simulink model "untitled"  (R2022a)
settings: Solver=FixedStepDiscrete  StartTime=0.0  StopTime=10.0  FixedStep=0.001  RelTol=1e-3
undefined symbols (not defined in the file): DiscIntNeverNeededParam
libraries: GPIO_Lib x8, TIMERS_Lib x8, CAN_Lib x7, USART_Lib x3, STM32_Config_Lib x1
settings Model: Creator=Administrator  LastModifiedBy=Administrator
settings SolverCC: AutoInsertRateTranBlk=on
settings OptimizationCC: DefaultParameterBehavior=Inlined  EnhancedBackFolding=on  PassReuseOutputArgsAs=Individual arguments  ZeroExternalMemoryAtStartup=off  ZeroInternalMemoryAtStartup=off  OptimizeBlockOrder=speed  DifferentSizesBufferReuse=on  OptimizationCustomize=off  EfficientTunableParamExpr=on
settings DebuggingCC: MultiTaskDSMMsg=none  ParameterTunabilityLossMsg=error
settings HardwareCC: ProdBitPerPointer=32  ProdBitPerSizeT=32  ProdBitPerPtrDiffT=32  ProdLargestAtomicInteger=Long  ProdLargestAtomicFloat=Double  ProdWordSize=32  ProdHWDeviceType=ARM Compatible->ARM Cortex-M
settings SFSimCC: MATLABDynamicMemAlloc=off
settings RTWCC: Description=stm32 (Embedded Target)  SystemTargetFile=stm32.tlc  TemplateMakefile=stm32.tmf  GenerateReport=on
settings RTWCC: CustomHeaderCode=|
  | #include "untitled_private.h"
  | #include "string.h"
  | #include "math.h"
settings CodeAppCC: ForceParamTrailComments=on  IgnoreCustomStorageClasses=off  MaxIdLength=64  OperatorAnnotations=on  SimulinkDataObjDesc=on  SFDataObjDesc=on  CustomSymbolStrType=$N$R$M  SimulinkBlockComments=off
settings STFCustomTargetCC: TargetLangStandard=C99 (ISO)  CodeReplacementLibrary=ARM CMSIS SIN COS  MultiwordLength=256  ParMdlRefBuildCompliant=on  IncludeMdlTerminateFcn=off  CombineOutputUpdateFcns=on  ERTCustomFileBanners=on  SupportNonInlinedSFcns=off  RemoveResetFunc=on  MATLABClassNameForMDSCustomization=Simulink.SoftwareTarget.ERTCustomization  GRTInterface=off  SystemTargetFile=stm32.tlc
settings ERTTargetCC: TargetLangStandard=C99 (ISO)  CodeReplacementLibrary=ARM CMSIS SIN COS  CompOptLevelCompliant=off  ConcurrentExecutionCompliant=off  IncludeMdlTerminateFcn=off  SupportContinuousTime=on  ModelStepFunctionPrototypeControlCompliant=off  CPPClassGenCompliant=off  UseToolchainInfoCompliant=off  ExtModeStaticAllocSize=256  ExtModeMexFile=ext_serial_win32_comm  ExtModeMexArgs=0,1,115200,10  InlinedParameterPlacement=NonHierarchical  ERTSrcFileBannerTemplate=sourceFileTemplate.cgt  ERTHdrFileBannerTemplate=sourceFileTemplate.cgt  ERTDataSrcFileTemplate=sourceFileTemplate.cgt  ERTDataHdrFileTemplate=sourceFileTemplate.cgt  ERTCustomFileTemplate=customRoutineProcess.tlc

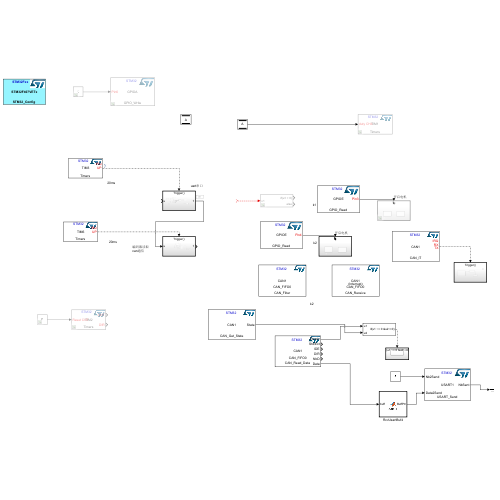
[thumbnail: Simulink's stored preview of the top-level diagram]
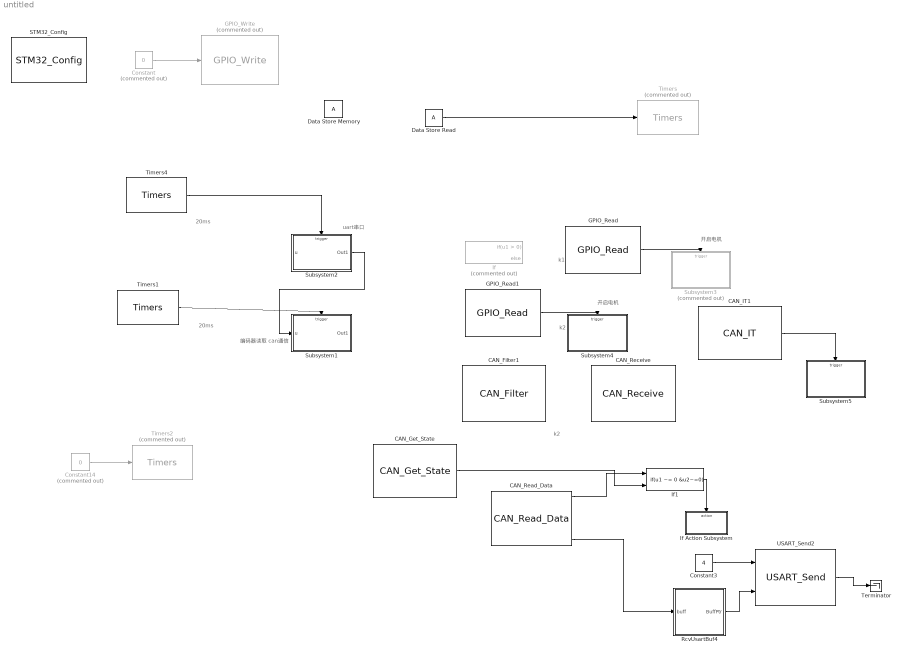
== system untitled ==
  note: 开启电机
  note: uart串口
  note: 编码器读取
      | can通信
  note: 20ms
  note: 20ms
  note: k2
  note: k1
  note: k2
  note: 开启电机
  CAN_Filter1 : CAN_Lib/CAN_Filter  CAN_name=CAN1  CAN_Filter_Activation=on  CAN_Filter_Scale=CAN_FILTERSCALE_16BIT  CAN_Filter_Mask_Id_High=0  CAN_Filter_Mask_Id_Low=0  CAN_Filter_Id_High=0  CAN_Filter_Id_Low=0  CAN_Filter_FIFO_Assignment=CAN_FIFO0  CAN_Filter_Bank=0  CAN_Filter_Mode=CAN_FILTERMODE_IDMASK  CAN_Filter_Slave_Start_Bank=14
      settings: SourceProductName=Target Support Package - STM32 Adapter
  CAN_Get_State : CAN_Lib/CAN_Get_State  CAN_name=CAN1
      settings: SourceProductName=Target Support Package - STM32 Adapter
  CAN_IT1 : CAN_Lib/CAN_IT  CAN_name=CAN1  CAN_Mode=Master  CAN_It=on  CAN_RX_It=on  CAN_TX_It=on  CAN_ERROR_It=off
      settings: SourceProductName=Target Support Package - STM32 Adapter
  CAN_Read_Data : CAN_Lib/CAN_Read_Data  CAN_name=CAN1  CAN_Fifo=CAN_FIFO0  CAN_MsgType=off
      settings: SourceProductName=Target Support Package - STM32 Adapter
  CAN_Receive : CAN_Lib/CAN_Receive  CAN_name=CAN1  CAN_Mode=Master  CAN_It=on  CAN_Fifo=CAN_FIFO0
      settings: SourceProductName=Target Support Package - STM32 Adapter
  Constant : Constant  Commented=on  Value=0
  Constant14 : Constant  Commented=on  Value=0  OutDataTypeStr=uint16
  Constant3 : Constant  Value=4  OutDataTypeStr=uint16
  Data Store Memory : DataStoreMemory  WriteAfterWriteMsg=warning  ShowAdditionalParam=off
  Data Store Read : DataStoreRead  IndexOptions=Index vector (dialog)  Indices=1  OutputSizes=1
  GPIO_Read : GPIO_Lib/GPIO_Read  Port_name=GPIOE  Pin_0=off  Pin_1=off  Pin_2=off  Pin_3=on  Pin_4=off  Pin_5=off  Pin_6=off  Pin_7=off  Pin_8=off  Pin_9=off  Pin_10=off  Pin_11=off  Pin_12=off  Pin_13=off  Pin_14=off  Pin_15=off  PinList="GPIOE3  4"
      settings: SourceProductName=Target Support Package - STM32 Adapter
  GPIO_Read1 : GPIO_Lib/GPIO_Read  Port_name=GPIOE  Pin_0=off  Pin_1=off  Pin_2=off  Pin_3=off  Pin_4=on  Pin_5=off  Pin_6=off  Pin_7=off  Pin_8=off  Pin_9=off  Pin_10=off  Pin_11=off  Pin_12=off  Pin_13=off  Pin_14=off  Pin_15=off  PinList="GPIOE3  4"
      settings: SourceProductName=Target Support Package - STM32 Adapter
  GPIO_Write : GPIO_Lib/GPIO_Write  Commented=on  Port_name=GPIOA  Pin0=off  Toggle_Pin0=off  Pin1=off  Toggle_Pin1=off  Pin2=off  Toggle_Pin2=off  Pin3=off  Toggle_Pin3=off  Pin4=off  Toggle_Pin4=off  Pin5=off  Toggle_Pin5=off  Pin6=on  Toggle_Pin6=off  Pin7=off  Toggle_Pin7=off  Pin8=off  Toggle_Pin8=off  Pin9=off  Toggle_Pin9=off  Pin10=off  Toggle_Pin10=off  Pin11=off  Toggle_Pin11=off  Pin12=off  Toggle_Pin12=off  Pin13=off  Toggle_Pin13=off  Pin14=off  Toggle_Pin14=off  Pin15=off  Toggle_Pin15=off  PinList="GPIOA6  7GPIOE13"
      settings: SourceProductName=Target Support Package - STM32 Adapter
  If : If  Commented=on
  If Action Subsystem : Subsystem  TreatAsAtomicUnit=on
  If1 : If  NumInputs=2  IfExpression=u1 ~= 0 &u2~=0  ShowElse=off
  RcvUsartBuf4 : MATLAB Function  TreatAsAtomicUnit=on
  STM32_Config : STM32_Config_Lib/STM32_Config  Priority=0  Project_Path=C:\Users\Administrator\Desktop\bishe\  Config_File=bishe.ioc  MCU_Name=STM32F407VETx
      settings: SourceProductName=Target Support Package - STM32 Adapter
  Subsystem1 : Subsystem
  Subsystem2 : Subsystem
  Subsystem3 : Subsystem  Commented=on
  Subsystem4 : Subsystem
  Subsystem5 : Subsystem
  Terminator : Terminator
  Timers : TIMERS_Lib/Timers  Commented=on  currentTIM=TIM1  TIM_Name=TIM1  sysUsingTimer=off  TIM_APBClock=168000000  TIM_Set_Clk=off  TIM_Prescaler=1000-1  TIM_Clock=168000.00  Variable_frequency=off  TIM_Set_OutFreq=off  TIM_ARR=1  Output_frequency=168000.00  Repetition_counter=0  TIM_Mode=Up  TIM_DMA=none  TIM_IRQ=on  TIM_IRQ_ONLY=off  TIM_UP=off  TIM_TRG=off  TIM_COM=off  TIM_BRK=off  NbTIM=5  CH1_enable=off  CH1N_enable=off  CH1_type=Unknown  CH1_DMA=off  CH1_int=off  CH1_edge=Rising  CH1_div=1  CH1_variable_duty=off  CH1_set_pulse=off  CH1_output_duty=0.00  CH1_pulse=0  CH2_enable=off  CH2N_enable=off  CH2_type=Unknown  CH2_DMA=off  CH2_int=off  CH2_edge=Rising  CH2_div=1  CH2_variable_duty=off  CH2_set_pulse=off  CH2_output_duty=0.00  CH2_pulse=0  CH3_enable=off  CH3N_enable=off  CH3_type=Unknown  CH3_DMA=off  CH3_int=off  CH3_edge=Rising  CH3_div=1  CH3_variable_duty=off  CH3_set_pulse=off  CH3_output_duty=0.00  CH3_pulse=0  CH4_enable=on  CH4N_enable=off  CH4_type=Output_PWM  CH4_DMA=off  CH4_int=off  CH4_edge=Rising  CH4_div=1  CH4_variable_duty=on  CH4_set_pulse=on  CH4_output_duty=0.00  CH4_pulse=0
      settings: SourceProductName=Target Support Package - STM32 Adapter
  Timers1 : TIMERS_Lib/Timers  currentTIM=TIM6  TIM_Name=TIM6  sysUsingTimer=off  TIM_APBClock=84000000  TIM_Set_Clk=off  TIM_Prescaler=8399  TIM_Clock=10000.00  Variable_frequency=off  TIM_Set_OutFreq=on  TIM_ARR=200  Output_frequency=50.00  Repetition_counter=0  TIM_Mode=Up  TIM_DMA=none  TIM_IRQ=off  TIM_IRQ_ONLY=on  TIM_UP=on  TIM_TRG=off  TIM_COM=off  TIM_BRK=off  NbTIM=5  CH1_enable=off  CH1N_enable=off  CH1_type=Unknown  CH1_DMA=off  CH1_int=off  CH1_edge=Rising  CH1_div=1  CH1_variable_duty=off  CH1_set_pulse=off  CH1_output_duty=0.00  CH1_pulse=0  CH2_enable=off  CH2N_enable=off  CH2_type=Unknown  CH2_DMA=off  CH2_int=off  CH2_edge=Rising  CH2_div=1  CH2_variable_duty=off  CH2_set_pulse=off  CH2_output_duty=0.00  CH2_pulse=0  CH3_enable=off  CH3N_enable=off  CH3_type=Unknown  CH3_DMA=off  CH3_int=off  CH3_edge=Rising  CH3_div=1  CH3_variable_duty=off  CH3_set_pulse=off  CH3_output_duty=0.00  CH3_pulse=0  CH4_enable=off  CH4N_enable=off  CH4_type=Unknown  CH4_DMA=off  CH4_int=off  CH4_edge=Rising  CH4_div=1  CH4_variable_duty=off  CH4_set_pulse=off  CH4_output_duty=0.00  CH4_pulse=0
      settings: SourceProductName=Target Support Package - STM32 Adapter
  Timers2 : TIMERS_Lib/Timers  Commented=on  currentTIM=TIM2  TIM_Name=TIM2  sysUsingTimer=off  TIM_APBClock=84000000  TIM_Set_Clk=off  TIM_Prescaler=3  TIM_Clock=21000000.00  Variable_frequency=off  TIM_Set_OutFreq=off  TIM_ARR=65535  Output_frequency=320.44  Repetition_counter=0  TIM_Mode=Up  TIM_DMA=none  TIM_IRQ=on  TIM_IRQ_ONLY=off  TIM_UP=off  TIM_TRG=off  TIM_COM=off  TIM_BRK=off  NbTIM=5  CH1_enable=on  CH1N_enable=off  CH1_type=Input_Encoder  CH1_DMA=off  CH1_int=off  CH1_edge=Rising  CH1_div=1  CH1_variable_duty=off  CH1_set_pulse=off  CH1_output_duty=0.00  CH1_pulse=0  CH2_enable=on  CH2N_enable=off  CH2_type=Input_Encoder  CH2_DMA=off  CH2_int=off  CH2_edge=Rising  CH2_div=1  CH2_variable_duty=off  CH2_set_pulse=off  CH2_output_duty=0.00  CH2_pulse=0  CH3_enable=off  CH3N_enable=off  CH3_type=Unknown  CH3_DMA=off  CH3_int=off  CH3_edge=Rising  CH3_div=1  CH3_variable_duty=off  CH3_set_pulse=off  CH3_output_duty=0.00  CH3_pulse=0  CH4_enable=off  CH4N_enable=off  CH4_type=Unknown  CH4_DMA=off  CH4_int=off  CH4_edge=Rising  CH4_div=1  CH4_variable_duty=off  CH4_set_pulse=off  CH4_output_duty=0.00  CH4_pulse=0
      settings: SourceProductName=Target Support Package - STM32 Adapter
  Timers4 : TIMERS_Lib/Timers  currentTIM=TIM3  TIM_Name=TIM3  sysUsingTimer=off  TIM_APBClock=84000000  TIM_Set_Clk=off  TIM_Prescaler=8399  TIM_Clock=10000.00  Variable_frequency=off  TIM_Set_OutFreq=on  TIM_ARR=100  Output_frequency=100.00  Repetition_counter=0  TIM_Mode=Up  TIM_DMA=none  TIM_IRQ=on  TIM_IRQ_ONLY=on  TIM_UP=on  TIM_TRG=off  TIM_COM=off  TIM_BRK=off  NbTIM=5  CH1_enable=off  CH1N_enable=off  CH1_type=Unknown  CH1_DMA=off  CH1_int=off  CH1_edge=Rising  CH1_div=1  CH1_variable_duty=off  CH1_set_pulse=off  CH1_output_duty=0.00  CH1_pulse=0  CH2_enable=off  CH2N_enable=off  CH2_type=Unknown  CH2_DMA=off  CH2_int=off  CH2_edge=Rising  CH2_div=1  CH2_variable_duty=off  CH2_set_pulse=off  CH2_output_duty=0.00  CH2_pulse=0  CH3_enable=off  CH3N_enable=off  CH3_type=Unknown  CH3_DMA=off  CH3_int=off  CH3_edge=Rising  CH3_div=1  CH3_variable_duty=off  CH3_set_pulse=off  CH3_output_duty=0.00  CH3_pulse=0  CH4_enable=off  CH4N_enable=off  CH4_type=Unknown  CH4_DMA=off  CH4_int=off  CH4_edge=Rising  CH4_div=1  CH4_variable_duty=off  CH4_set_pulse=off  CH4_output_duty=0.00  CH4_pulse=0
      settings: SourceProductName=Target Support Package - STM32 Adapter
  USART_Send2 : USART_Lib/USART_Send  USART_name=USART1  Buff_size=256  nbUsart=2  usartMode=Asynchronous  usartDma_Rx=off  usartDma_Tx=off  usartIt=on
      settings: SourceProductName=Target Support Package - STM32 Adapter
  wires:
  Constant/1 -> GPIO_Write/1
  Timers1/1 -> Subsystem1/Trigger
  Timers4/1 -> Subsystem2/Trigger
  GPIO_Read/1 -> Subsystem3/Trigger
  Constant14/1 -> Timers2/1
  Data Store Read/1 -> Timers/1
  Subsystem2/1(Out1) -> Subsystem1/1(u)
  ? -> If/1
  GPIO_Read1/1 -> Subsystem4/Trigger
  CAN_IT1/1 -> Subsystem5/Trigger
  CAN_Read_Data/1 -> If1/1
  CAN_Get_State/1 -> If1/2
  If1/1 -> If Action Subsystem/Action
  Constant3/1 -> USART_Send2/1
  RcvUsartBuf4/1(BuffPtr) -> USART_Send2/2
  USART_Send2/1 -> Terminator/1
  CAN_Read_Data/6 -> RcvUsartBuf4/1(buff)

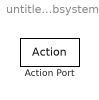
== system untitled/If Action Subsystem ==
  Action Port : ActionPort  ActionPortLabel=if(u1 ~= 0 &u2~=0)

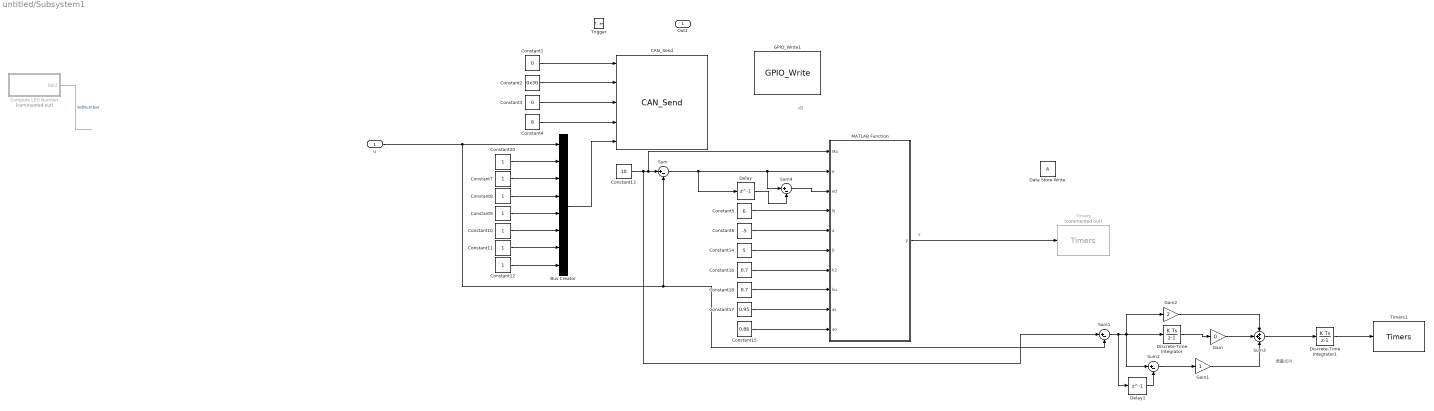
== system untitled/Subsystem1 ==
  note: 增量式PI
  note: y
  note: d2
  u : Inport
  Trigger : TriggerPort  TriggerType=function-call  VariantControl=(inherit)  PortDimensions=1
  Bus Creator : BusCreator  Inputs=8
  CAN_Send : CAN_Lib/CAN_Send  CAN_name=CAN1  CAN_Mode=Master  CAN_It=on  CAN_MsgType=off
      settings: SourceProductName=Target Support Package - STM32 Adapter
  Compute LED Number : Subsystem  Priority=21  Commented=on  TreatAsAtomicUnit=on  RTWFcnName=computeLedNumber
      settings: AttributesFormatString=Priority=%<Priority>  RTWFcnNameOpts=User specified
  Constant1 : Constant  Value=0  OutDataTypeStr=uint16
  Constant{7..12,20} (7 alike) : Constant  OutDataTypeStr=uint8
  Constant13 : Constant  Value=10  OutDataTypeStr=double
  Constant14 : Constant  Value=5  OutDataTypeStr=double
  Constant15 : Constant  Value=0.86  OutDataTypeStr=double
  Constant16 : Constant  Value=0.7  OutDataTypeStr=double
  Constant17 : Constant  Value=0.95  OutDataTypeStr=double
  Constant18 : Constant  Value=0.7  OutDataTypeStr=double
  Constant2 : Constant  Value=0x30  OutDataTypeStr=uint16
  Constant3 : Constant  Value=0  OutDataTypeStr=uint16
  Constant4 : Constant  Value=8  OutDataTypeStr=uint16
  Constant5 : Constant  Value=6  OutDataTypeStr=double
  Constant6 : Constant  Value=-5  OutDataTypeStr=double
  Data Store Write : DataStoreWrite  IndexOptions=Index vector (dialog)  Indices=1  OutputSizes=1
  Delay : Delay  DelayLength=1  InitialCondition=0
  Delay1 : Delay  DelayLength=1  InitialCondition=0
  Discrete-Time Integrator : DiscreteIntegrator  SampleTime=-1  ICPrevOutput=DiscIntNeverNeededParam  ICPrevScaledInput=DiscIntNeverNeededParam
  Discrete-Time Integrator1 : DiscreteIntegrator  SampleTime=-1  ICPrevOutput=DiscIntNeverNeededParam  ICPrevScaledInput=DiscIntNeverNeededParam
  GPIO_Write1 : GPIO_Lib/GPIO_Write  Port_name=GPIOA  Pin0=off  Toggle_Pin0=off  Pin1=off  Toggle_Pin1=off  Pin2=off  Toggle_Pin2=off  Pin3=off  Toggle_Pin3=off  Pin4=off  Toggle_Pin4=off  Pin5=off  Toggle_Pin5=off  Pin6=on  Toggle_Pin6=on  Pin7=off  Toggle_Pin7=off  Pin8=off  Toggle_Pin8=off  Pin9=off  Toggle_Pin9=off  Pin10=off  Toggle_Pin10=off  Pin11=off  Toggle_Pin11=off  Pin12=off  Toggle_Pin12=off  Pin13=off  Toggle_Pin13=off  Pin14=off  Toggle_Pin14=off  Pin15=off  Toggle_Pin15=off  PinList="GPIOA6  7GPIOE13"
      settings: SourceProductName=Target Support Package - STM32 Adapter
  Gain : Gain  Gain=0
  Gain1 : Gain
  Gain2 : Gain  Gain=2
  MATLAB Function : MATLAB Function  TreatAsAtomicUnit=on
  Sum{,1..2,4} (4 alike) : Sum  Inputs=|+-
  Sum3 : Sum  Inputs=+++
  Timers : TIMERS_Lib/Timers  Commented=on  currentTIM=TIM1  TIM_Name=TIM1  sysUsingTimer=off  TIM_APBClock=168000000  TIM_Set_Clk=off  TIM_Prescaler=167  TIM_Clock=1000000.00  Variable_frequency=off  TIM_Set_OutFreq=on  TIM_ARR=1000  Output_frequency=1000.00  Repetition_counter=0  TIM_Mode=Up  TIM_DMA=none  TIM_IRQ=on  TIM_IRQ_ONLY=off  TIM_UP=off  TIM_TRG=off  TIM_COM=off  TIM_BRK=off  NbTIM=5  CH1_enable=off  CH1N_enable=off  CH1_type=Unknown  CH1_DMA=off  CH1_int=off  CH1_edge=Rising  CH1_div=1  CH1_variable_duty=off  CH1_set_pulse=off  CH1_output_duty=0.00  CH1_pulse=0  CH2_enable=off  CH2N_enable=off  CH2_type=Unknown  CH2_DMA=off  CH2_int=off  CH2_edge=Rising  CH2_div=1  CH2_variable_duty=off  CH2_set_pulse=off  CH2_output_duty=0.00  CH2_pulse=0  CH3_enable=off  CH3N_enable=off  CH3_type=Output_PWM  CH3_DMA=off  CH3_int=off  CH3_edge=Rising  CH3_div=1  CH3_variable_duty=off  CH3_set_pulse=on  CH3_output_duty=10.00  CH3_pulse=100  CH4_enable=on  CH4N_enable=off  CH4_type=Output_PWM  CH4_DMA=off  CH4_int=off  CH4_edge=Rising  CH4_div=1  CH4_variable_duty=on  CH4_set_pulse=off  CH4_output_duty=5.00  CH4_pulse=50
      settings: SourceProductName=Target Support Package - STM32 Adapter
  Timers1 : TIMERS_Lib/Timers  currentTIM=TIM1  TIM_Name=TIM1  sysUsingTimer=off  TIM_APBClock=168000000  TIM_Set_Clk=off  TIM_Prescaler=167  TIM_Clock=1000000.00  Variable_frequency=off  TIM_Set_OutFreq=on  TIM_ARR=1000  Output_frequency=1000.00  Repetition_counter=0  TIM_Mode=Up  TIM_DMA=none  TIM_IRQ=on  TIM_IRQ_ONLY=off  TIM_UP=off  TIM_TRG=off  TIM_COM=off  TIM_BRK=off  NbTIM=5  CH1_enable=off  CH1N_enable=off  CH1_type=Unknown  CH1_DMA=off  CH1_int=off  CH1_edge=Rising  CH1_div=1  CH1_variable_duty=off  CH1_set_pulse=off  CH1_output_duty=0.00  CH1_pulse=0  CH2_enable=off  CH2N_enable=off  CH2_type=Unknown  CH2_DMA=off  CH2_int=off  CH2_edge=Rising  CH2_div=1  CH2_variable_duty=off  CH2_set_pulse=off  CH2_output_duty=0.00  CH2_pulse=0  CH3_enable=off  CH3N_enable=off  CH3_type=Output_PWM  CH3_DMA=off  CH3_int=off  CH3_edge=Rising  CH3_div=1  CH3_variable_duty=off  CH3_set_pulse=on  CH3_output_duty=10.00  CH3_pulse=100  CH4_enable=on  CH4N_enable=off  CH4_type=Output_PWM  CH4_DMA=off  CH4_int=off  CH4_edge=Rising  CH4_div=1  CH4_variable_duty=on  CH4_set_pulse=off  CH4_output_duty=5.00  CH4_pulse=50
      settings: SourceProductName=Target Support Package - STM32 Adapter
  Out1 : Outport
  wires:
  Constant1/1 -> CAN_Send/1
  Constant2/1 -> CAN_Send/2
  Constant3/1 -> CAN_Send/3
  Constant4/1 -> CAN_Send/4
  Bus Creator/1 -> CAN_Send/5
  Constant8/1 -> Bus Creator/4
  Constant7/1 -> Bus Creator/3
  Constant12/1 -> Bus Creator/8
  Constant11/1 -> Bus Creator/7
  Constant10/1 -> Bus Creator/6
  Constant9/1 -> Bus Creator/5
  Compute LED Number/1(Out2) -> ?  "ledNumber"
  u/1 -> Sum1/2, Sum/2, Bus Creator/1
  Sum/1 -> Sum4/1, MATLAB Function/2(e), Delay/1
  Constant13/1 -> Sum1/1, MATLAB Function/1(Ma), Sum/1
  Constant5/1 -> MATLAB Function/4(N)
  Constant6/1 -> MATLAB Function/5(a)
  Constant14/1 -> MATLAB Function/6(b)
  Constant15/1 -> MATLAB Function/10(ao)
  Constant16/1 -> MATLAB Function/7(k2)
  Constant17/1 -> MATLAB Function/9(as)
  Constant18/1 -> MATLAB Function/8(ku)
  Constant20/1 -> Bus Creator/2
  Sum1/1 -> Delay1/1, Discrete-Time Integrator/1, Sum2/1, Gain2/1
  Discrete-Time Integrator/1 -> Gain/1
  Gain1/1 -> Sum3/3
  Gain/1 -> Sum3/2
  Gain2/1 -> Sum3/1
  Delay1/1 -> Sum2/2
  Sum2/1 -> Gain1/1
  Discrete-Time Integrator1/1 -> Timers1/1
  Sum3/1 -> Discrete-Time Integrator1/1
  MATLAB Function/1(y) -> Timers/1
  Delay/1 -> Sum4/2
  Sum4/1 -> MATLAB Function/3(ed)

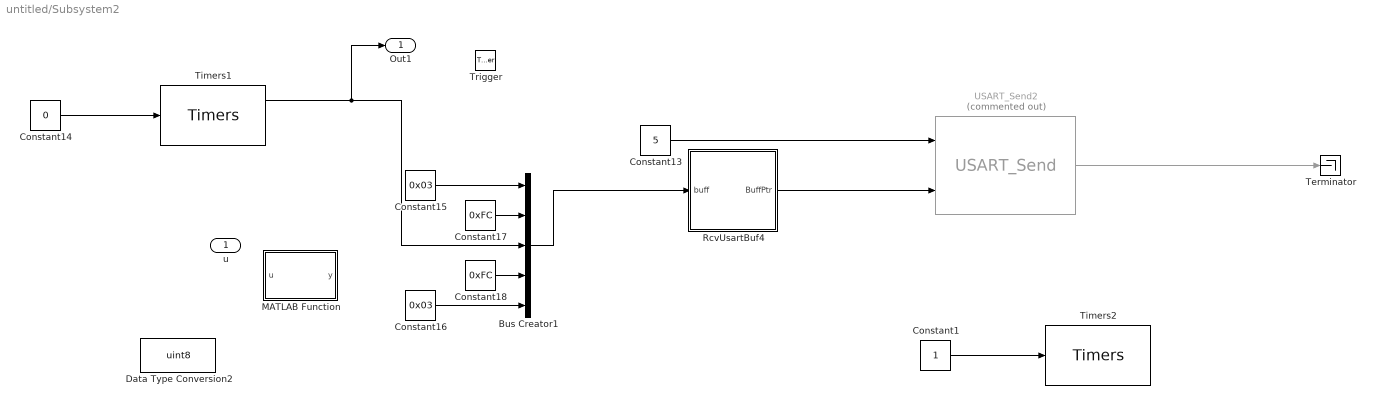
== system untitled/Subsystem2 ==
  u : Inport
  Trigger : TriggerPort  TriggerType=function-call  VariantControl=(inherit)  PortDimensions=1
  Bus Creator1 : BusCreator  Inputs=5
  Constant1 : Constant  OutDataTypeStr=uint16
  Constant13 : Constant  Value=5  OutDataTypeStr=uint16
  Constant14 : Constant  Value=0  OutDataTypeStr=uint16
  Constant15 : Constant  Value=0x03  OutDataTypeStr=uint8
  Constant16 : Constant  Value=0x03  OutDataTypeStr=uint8
  Constant17 : Constant  Value=0xFC  OutDataTypeStr=uint8
  Constant18 : Constant  Value=0xFC  OutDataTypeStr=uint8
  Data Type Conversion2 : DataTypeConversion  OutMin=[0]  OutMax=[255]  OutDataTypeStr=uint8  SaturateOnIntegerOverflow=off  RndMeth=Floor
  MATLAB Function : MATLAB Function  TreatAsAtomicUnit=on
  RcvUsartBuf4 : MATLAB Function  TreatAsAtomicUnit=on
  Terminator : Terminator
  Timers1 : TIMERS_Lib/Timers  currentTIM=TIM2  TIM_Name=TIM2  sysUsingTimer=off  TIM_APBClock=84000000  TIM_Set_Clk=off  TIM_Prescaler=3  TIM_Clock=21000000.00  Variable_frequency=off  TIM_Set_OutFreq=off  TIM_ARR=2100  Output_frequency=10000.00  Repetition_counter=0  TIM_Mode=Up  TIM_DMA=none  TIM_IRQ=on  TIM_IRQ_ONLY=off  TIM_UP=off  TIM_TRG=off  TIM_COM=off  TIM_BRK=off  NbTIM=5  CH1_enable=on  CH1N_enable=off  CH1_type=Input_Encoder  CH1_DMA=off  CH1_int=off  CH1_edge=Rising  CH1_div=1  CH1_variable_duty=off  CH1_set_pulse=off  CH1_output_duty=0.00  CH1_pulse=0  CH2_enable=on  CH2N_enable=off  CH2_type=Input_Encoder  CH2_DMA=off  CH2_int=off  CH2_edge=Rising  CH2_div=1  CH2_variable_duty=off  CH2_set_pulse=off  CH2_output_duty=0.00  CH2_pulse=0  CH3_enable=off  CH3N_enable=off  CH3_type=Unknown  CH3_DMA=off  CH3_int=off  CH3_edge=Rising  CH3_div=1  CH3_variable_duty=off  CH3_set_pulse=off  CH3_output_duty=0.00  CH3_pulse=0  CH4_enable=off  CH4N_enable=off  CH4_type=Unknown  CH4_DMA=off  CH4_int=off  CH4_edge=Rising  CH4_div=1  CH4_variable_duty=off  CH4_set_pulse=off  CH4_output_duty=0.00  CH4_pulse=0
      settings: SourceProductName=Target Support Package - STM32 Adapter
  Timers2 : TIMERS_Lib/Timers  currentTIM=TIM2  TIM_Name=TIM2  sysUsingTimer=off  TIM_APBClock=84000000  TIM_Set_Clk=off  TIM_Prescaler=3  TIM_Clock=21000000.00  Variable_frequency=off  TIM_Set_OutFreq=off  TIM_ARR=2100  Output_frequency=10000.00  Repetition_counter=0  TIM_Mode=Up  TIM_DMA=none  TIM_IRQ=on  TIM_IRQ_ONLY=off  TIM_UP=off  TIM_TRG=off  TIM_COM=off  TIM_BRK=off  NbTIM=5  CH1_enable=on  CH1N_enable=off  CH1_type=Input_Encoder  CH1_DMA=off  CH1_int=off  CH1_edge=Rising  CH1_div=1  CH1_variable_duty=off  CH1_set_pulse=off  CH1_output_duty=0.00  CH1_pulse=0  CH2_enable=on  CH2N_enable=off  CH2_type=Input_Encoder  CH2_DMA=off  CH2_int=off  CH2_edge=Rising  CH2_div=1  CH2_variable_duty=off  CH2_set_pulse=off  CH2_output_duty=0.00  CH2_pulse=0  CH3_enable=off  CH3N_enable=off  CH3_type=Unknown  CH3_DMA=off  CH3_int=off  CH3_edge=Rising  CH3_div=1  CH3_variable_duty=off  CH3_set_pulse=off  CH3_output_duty=0.00  CH3_pulse=0  CH4_enable=off  CH4N_enable=off  CH4_type=Unknown  CH4_DMA=off  CH4_int=off  CH4_edge=Rising  CH4_div=1  CH4_variable_duty=off  CH4_set_pulse=off  CH4_output_duty=0.00  CH4_pulse=0
      settings: SourceProductName=Target Support Package - STM32 Adapter
  USART_Send2 : USART_Lib/USART_Send  Commented=on  USART_name=USART1  Buff_size=256  nbUsart=2  usartMode=Asynchronous  usartDma_Rx=off  usartDma_Tx=off  usartIt=on
      settings: SourceProductName=Target Support Package - STM32 Adapter
  Out1 : Outport
  wires:
  Constant16/1 -> Bus Creator1/5
  Constant18/1 -> Bus Creator1/4
  USART_Send2/1 -> Terminator/1
  Bus Creator1/1 -> RcvUsartBuf4/1(buff)
  Constant17/1 -> Bus Creator1/2
  RcvUsartBuf4/1(BuffPtr) -> USART_Send2/2
  Constant13/1 -> USART_Send2/1
  Constant15/1 -> Bus Creator1/1
  Constant14/1 -> Timers1/1
  Constant1/1 -> Timers2/1
  Timers1/1 -> Out1/1, Bus Creator1/3

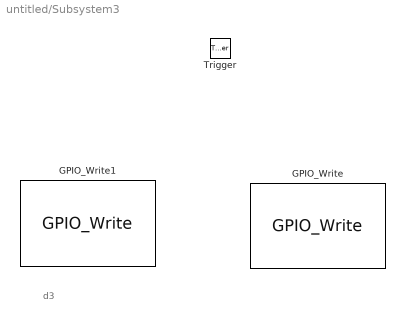
== system untitled/Subsystem3 ==
  note: d3
  Trigger : TriggerPort  TriggerType=falling  VariantControl=(inherit)  PortDimensions=1
  GPIO_Write : GPIO_Lib/GPIO_Write  Port_name=GPIOE  Pin0=off  Toggle_Pin0=off  Pin1=off  Toggle_Pin1=off  Pin2=off  Toggle_Pin2=off  Pin3=off  Toggle_Pin3=off  Pin4=off  Toggle_Pin4=off  Pin5=off  Toggle_Pin5=off  Pin6=off  Toggle_Pin6=off  Pin7=off  Toggle_Pin7=off  Pin8=off  Toggle_Pin8=off  Pin9=off  Toggle_Pin9=off  Pin10=off  Toggle_Pin10=off  Pin11=off  Toggle_Pin11=off  Pin12=off  Toggle_Pin12=off  Pin13=on  Toggle_Pin13=on  Pin14=off  Toggle_Pin14=off  Pin15=off  Toggle_Pin15=off  PinList="GPIOA6  7GPIOE13"
      settings: SourceProductName=Target Support Package - STM32 Adapter
  GPIO_Write1 : GPIO_Lib/GPIO_Write  Port_name=GPIOA  Pin0=off  Toggle_Pin0=off  Pin1=off  Toggle_Pin1=off  Pin2=off  Toggle_Pin2=off  Pin3=off  Toggle_Pin3=off  Pin4=off  Toggle_Pin4=off  Pin5=off  Toggle_Pin5=off  Pin6=off  Toggle_Pin6=off  Pin7=on  Toggle_Pin7=on  Pin8=off  Toggle_Pin8=off  Pin9=off  Toggle_Pin9=off  Pin10=off  Toggle_Pin10=off  Pin11=off  Toggle_Pin11=off  Pin12=off  Toggle_Pin12=off  Pin13=off  Toggle_Pin13=off  Pin14=off  Toggle_Pin14=off  Pin15=off  Toggle_Pin15=off  PinList="GPIOA6  7GPIOE13"
      settings: SourceProductName=Target Support Package - STM32 Adapter

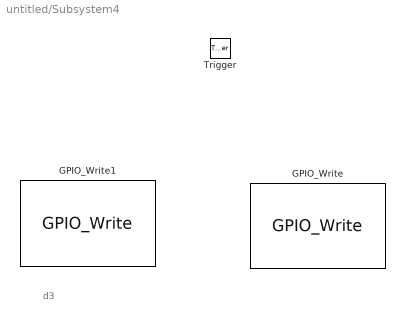
== system untitled/Subsystem4 ==
  note: d3
  Trigger : TriggerPort  TriggerType=falling  VariantControl=(inherit)  PortDimensions=1
  GPIO_Write : GPIO_Lib/GPIO_Write  Port_name=GPIOE  Pin0=off  Toggle_Pin0=off  Pin1=off  Toggle_Pin1=off  Pin2=off  Toggle_Pin2=off  Pin3=off  Toggle_Pin3=off  Pin4=off  Toggle_Pin4=off  Pin5=off  Toggle_Pin5=off  Pin6=off  Toggle_Pin6=off  Pin7=off  Toggle_Pin7=off  Pin8=off  Toggle_Pin8=off  Pin9=off  Toggle_Pin9=off  Pin10=off  Toggle_Pin10=off  Pin11=off  Toggle_Pin11=off  Pin12=off  Toggle_Pin12=off  Pin13=on  Toggle_Pin13=on  Pin14=off  Toggle_Pin14=off  Pin15=off  Toggle_Pin15=off  PinList="GPIOA6  7GPIOE13"
      settings: SourceProductName=Target Support Package - STM32 Adapter
  GPIO_Write1 : GPIO_Lib/GPIO_Write  Port_name=GPIOA  Pin0=off  Toggle_Pin0=off  Pin1=off  Toggle_Pin1=off  Pin2=off  Toggle_Pin2=off  Pin3=off  Toggle_Pin3=off  Pin4=off  Toggle_Pin4=off  Pin5=off  Toggle_Pin5=off  Pin6=off  Toggle_Pin6=off  Pin7=on  Toggle_Pin7=on  Pin8=off  Toggle_Pin8=off  Pin9=off  Toggle_Pin9=off  Pin10=off  Toggle_Pin10=off  Pin11=off  Toggle_Pin11=off  Pin12=off  Toggle_Pin12=off  Pin13=off  Toggle_Pin13=off  Pin14=off  Toggle_Pin14=off  Pin15=off  Toggle_Pin15=off  PinList="GPIOA6  7GPIOE13"
      settings: SourceProductName=Target Support Package - STM32 Adapter

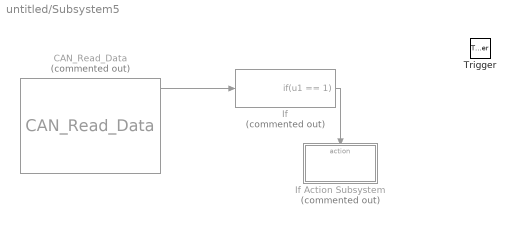
== system untitled/Subsystem5 ==
  Trigger : TriggerPort  TriggerType=function-call  VariantControl=(inherit)  PortDimensions=1
  CAN_Read_Data : CAN_Lib/CAN_Read_Data  Commented=on  CAN_name=CAN1  CAN_Fifo=CAN_FIFO0  CAN_MsgType=off
      settings: SourceProductName=Target Support Package - STM32 Adapter
  If : If  Commented=on  IfExpression=u1 == 1  ShowElse=off
  If Action Subsystem : Subsystem  Commented=on  TreatAsAtomicUnit=on
  wires:
  CAN_Read_Data/1 -> If/1
  If/1 -> If Action Subsystem/Action

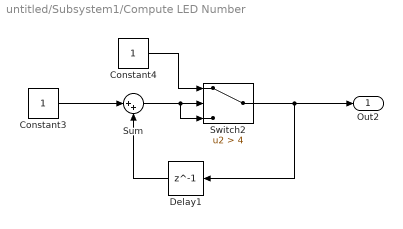
== system untitled/Subsystem1/Compute LED Number ==
  Constant3 : Constant  OutDataTypeStr=uint8
  Constant4 : Constant  OutDataTypeStr=uint8
  Delay1 : Delay  DelayLength=1  InitialCondition=0
  Sum : Sum  Inputs=|++
  Switch2 : Switch  Criteria=u2 > Threshold  Threshold=4  OutDataTypeStr=uint8  SaturateOnIntegerOverflow=off  InputSameDT=off
  Out2 : Outport  VectorParamsAs1DForOutWhenUnconnected=off
  wires:
  Sum/1 -> Switch2/3, Switch2/2
  Constant4/1 -> Switch2/1
  Delay1/1 -> Sum/2
  Constant3/1 -> Sum/1
  Switch2/1 -> Delay1/1, Out2/1

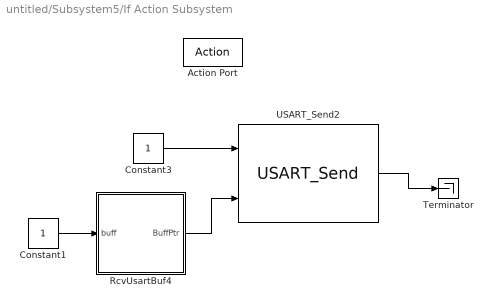
== system untitled/Subsystem5/If Action Subsystem ==
  Action Port : ActionPort  ActionPortLabel=if(u1 == 1)
  Constant1 : Constant  OutDataTypeStr=uint16
  Constant3 : Constant  OutDataTypeStr=uint16
  RcvUsartBuf4 : MATLAB Function  TreatAsAtomicUnit=on
  Terminator : Terminator
  USART_Send2 : USART_Lib/USART_Send  USART_name=USART1  Buff_size=256  nbUsart=1  usartMode=Asynchronous  usartDma_Rx=off  usartDma_Tx=off  usartIt=on
      settings: SourceProductName=Target Support Package - STM32 Adapter
  wires:
  Constant1/1 -> RcvUsartBuf4/1(buff)
  Constant3/1 -> USART_Send2/1
  RcvUsartBuf4/1(BuffPtr) -> USART_Send2/2
  USART_Send2/1 -> Terminator/1

== matlab function untitled/Subsystem5/If Action Subsystem/RcvUsartBuf4 ==
  data: BuffPtr output uint32 size=1; buff input
function BuffPtr = convert(buff)
if coder.target('Sfun')
    % Executing in MATLAB, Buff is null
    BuffPtr = uint32(0);
    %NbChar = uint16(0);
else
    coder.cinclude('getBuffPtr.h');
    % Executing in the generated code.
    BuffPtr = coder.ceval('getBuffPtr',coder.rref(buff));
end
end

== matlab function untitled/Subsystem1/MATLAB Function ==
  data: Ma input; e input; ed input; N input; y output; a input; b input; k2 input; ku input; as input; ao input
function y = fcn(Ma,e,ed,N,a,b,k2,ku,as,ao)

E=-(2*N)*(e*k2-(a+b))/(b-a); 
E1=E;
EC=-(2*N)*(ed-(a+b))/(b-a);
EC1=270*EC;
a1=(1/N)*(as-ao)*abs(E1)+ao;
u1=-(a1*E1+(1-a1)*EC1)/2;
y=u1*ku*Ma;

end

== matlab function untitled/Subsystem2/MATLAB Function ==
  data: u input; y output
function y = chu(u)
y = uint8(u/256);
%y = uint8(u/256);

== matlab function untitled/Subsystem2/RcvUsartBuf4 ==
  data: BuffPtr output uint32 size=1; buff input
function BuffPtr = convert(buff)
if coder.target('Sfun')
    % Executing in MATLAB, Buff is null
    BuffPtr = uint32(0);
    %NbChar = uint16(0);
else
    coder.cinclude('getBuffPtr.h');
    % Executing in the generated code.
    BuffPtr = coder.ceval('getBuffPtr',coder.rref(buff));
end
end

== matlab function untitled/RcvUsartBuf4 ==
  data: BuffPtr output uint32 size=1; buff input
function BuffPtr = convert(buff)
if coder.target('Sfun')
    % Executing in MATLAB, Buff is null
    BuffPtr = uint32(0);
    %NbChar = uint16(0);
else
    coder.cinclude('getBuffPtr.h');
    % Executing in the generated code.
    BuffPtr = coder.ceval('getBuffPtr',coder.rref(buff));
end
end
